simulink model "fullmodel0000001"  (R2016a)
settings: Solver=VariableStepAuto  StartTime=0.0  StopTime=10.0  RelTol=1e-3
values from neighbouring files (symbols this model uses):
  B = [0 ... (first row only)    [ssmodel.m]    (also in ssmodel2.m)
  J = 2.8033e-5    (= 2.8033e-05)    [values.m]
undefined symbols (not defined in the file or in its folder): kb, kt, l, La, r, Ra
settings Model: Creator=The MathWorks, Inc.  LastModifiedBy=jack
settings DataIOCC: LimitDataPoints=on
settings DebuggingCC: AllowSymbolicDim=off
settings ModelReferenceCC: PropagateSignalLabelsOutOfModel=off
settings GRTTargetCC: GeneratePreprocessorConditionals=Use local settings

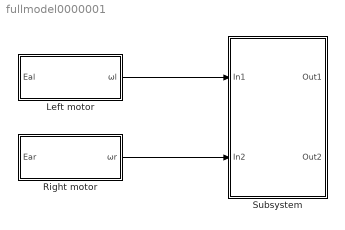
== system fullmodel0000001 ==
  Left motor : Subsystem
  Right motor : Subsystem
  Subsystem : Subsystem
  wires:
  Left motor/1(ωl) -> Subsystem/1(In1)
  Right motor/1(ωr) -> Subsystem/2(In2)
  ? -> Left motor/1(Eal)
  ? -> Right motor/1(Ear)

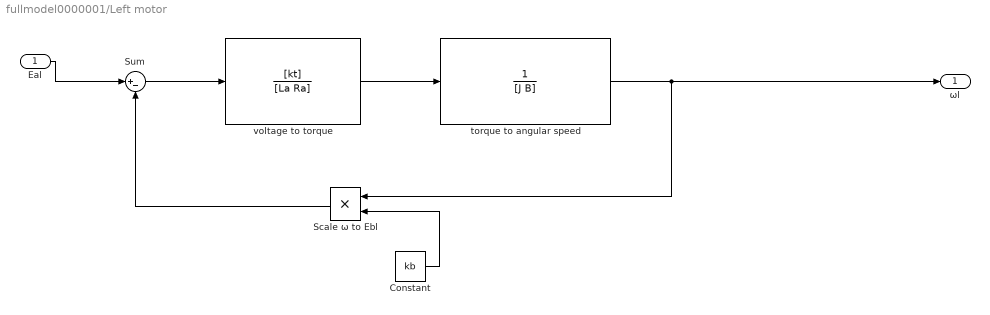
== system fullmodel0000001/Left motor ==
  Eal : Inport
  Constant : Constant  Value=kb
  Scale ω to Ebl : Product  Inputs=**
  Sum : Sum  Inputs=|+-
  torque to angular speed : TransferFcn  Denominator=[J B]
  voltage to torque : TransferFcn  Numerator=[kt]  Denominator=[La Ra]
  ωl : Outport
  wires:
  Eal/1 -> Sum/1
  Sum/1 -> voltage to torque/1
  voltage to torque/1 -> torque to angular speed/1
  Scale ω to Ebl/1 -> Sum/2
  torque to angular speed/1 -> Scale ω to Ebl/1, ωl/1
  Constant/1 -> Scale ω to Ebl/2

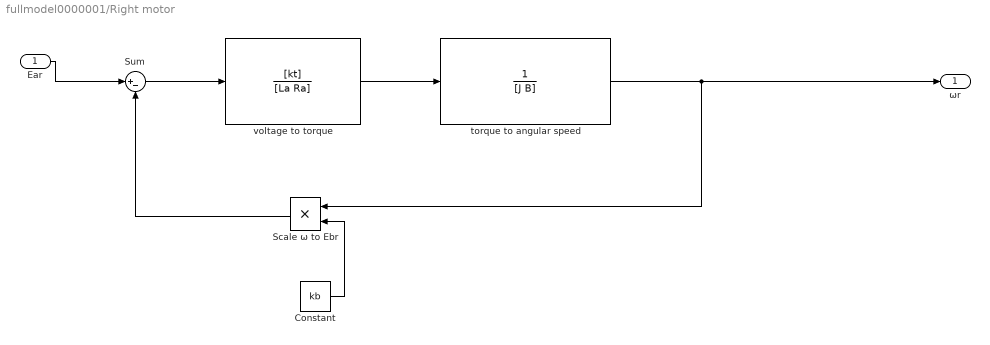
== system fullmodel0000001/Right motor ==
  Ear : Inport
  Constant : Constant  Value=kb
  Scale ω to Ebr : Product  Inputs=**
  Sum : Sum  Inputs=|+-
  torque to angular speed : TransferFcn  Denominator=[J B]
  voltage to torque : TransferFcn  Numerator=[kt]  Denominator=[La Ra]
  ωr : Outport
  wires:
  Sum/1 -> voltage to torque/1
  voltage to torque/1 -> torque to angular speed/1
  Ear/1 -> Sum/1
  Scale ω to Ebr/1 -> Sum/2
  torque to angular speed/1 -> Scale ω to Ebr/1, ωr/1
  Constant/1 -> Scale ω to Ebr/2

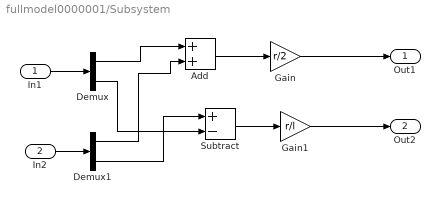
== system fullmodel0000001/Subsystem ==
  In1 : Inport
  In2 : Inport  Port=2
  Add : Sum
  Demux : Demux  Outputs=2
  Demux1 : Demux  Outputs=2
  Gain : Gain  Gain=r/2
  Gain1 : Gain  Gain=r/l
  Subtract : Sum  Inputs=+-
  Out1 : Outport
  Out2 : Outport  Port=2
  wires:
  In1/1 -> Demux/1
  In2/1 -> Demux1/1
  Demux/1 -> Add/1
  Demux1/1 -> Add/2
  Add/1 -> Gain/1
  Gain/1 -> Out1/1
  Demux1/2 -> Subtract/1
  Demux/2 -> Subtract/2
  Subtract/1 -> Gain1/1
  Gain1/1 -> Out2/1
